simulink model "wave_test_qpsk"  (R2017b)
settings: Solver=VariableStepAuto  StartTime=0.0  StopTime=10.0  RelTol=1e-3
undefined symbols (not defined in the file): ip, sdrqpsktx, usb
libraries: plutoradiolib x1, dspvision x1, plutoradioblksprivate x1, commutil2 x1, commdigbbndpm3 x1, commfilt2 x1
settings Model: Creator=root  LastModifiedBy=root

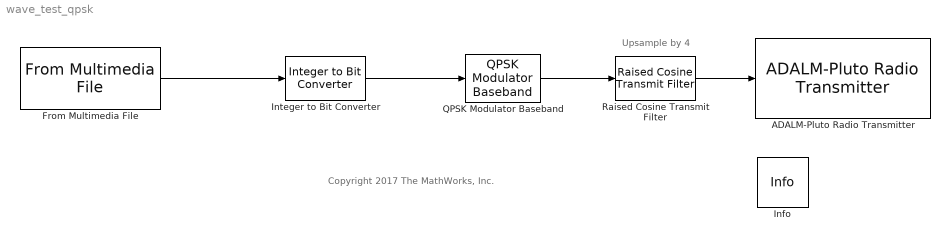
== system wave_test_qpsk ==
  note: Copyright 2017 The MathWorks, Inc.
  note: Upsample by 4
  ADALM-Pluto Radio Transmitter : plutoradiolib/ADALM-Pluto Radio Transmitter  SourceLibraryInfo="This block requires <a href=\"http://www.mathworks.com/hardware-support/rtl-sdr.html\">Communications System Toolbox Support Package for RTL-SDR Radio</a>"  RadioID=usb:0  uri=ip:10.0.0.200  CenterFrequencySource=Dialog  CenterFrequency=90.5e6  GainSource=Dialog  Gain=0  ChannelMapping=1  BasebandSampleRate=100e3  UnderflowOutputPort=off  ShowAdvancedProperties=off  Timeout=inf  DataSourceSelect=Input Port  DDSTone1Freq=5e3  DDSTone2Freq=10e3  DDSTone1Scale=0.5  DDSTone2Scale=0.25  FrequencyCorrection=0  UseCustomFilter=off  filtPathRates=[ 737280000, 11520000, 3840000, 1920000, 960000, 240000 ]  filtCoefficients=round( fir1( 127, 0.75 )*2^15*10^1.2 )  filtCoefficientSize=128  filtDecimInterpFactor=4  filtGain=-12  filtRFBandwidth=18e6  filterConfigStruct=struct()  ENSMPinControlMode=None  BISTLoopbackMode=Disabled
      settings: SourceProductName=Communications System Toolbox Support Package for ADALM-PLUTO Radio
  From Multimedia File : dspvision/From Multimedia File  inputFilename=/home/udsdrew/04_Let_Me_Be_Myself_mono.wav  loop=on  numPlays=inf  outputStreams=Audio only  videoDataType=single  audioDataType=int16  inheritSampleTime=on  userDefinedSampleTime=1/30  noAudioOutput=off  isIntensityVideo=off  fourcc=RGB  colorVideoFormat=One multidimensional signal  outputEOF=off  dataOrg=Column-major  audioFrameSize=8192  computeAudioFrameSize=off  outSamplingMode=Sample based
      settings: SourceProductBaseCode=VP
  Info : plutoradioblksprivate/Info  SystemSampleTime=-1
  Integer to Bit Converter : commutil2/Integer to Bit Converter  nbits=16  signedInputValues=Unsigned  bitOrder=MSB first  outDtype=Inherit via internal rule
  QPSK Modulator Baseband : commdigbbndpm3/QPSK Modulator Baseband  InType=Bit  Enc=Gray  Ph=pi/4  outDtype=double  outWordLen=16  outUDDataType=sfix(16)  outFracLenMode=Best precision  outFracLen=15  outDataTypeStr=double  outLastDataTypeStr=double
  Raised Cosine Transmit Filter : commfilt2/Raised Cosine Transmit Filter  filtType=Square root  R=sdrqpsktx.RollOff  filtSpan=sdrqpsktx.RCFiltSpan  N=sdrqpsktx.Upsampling  filterGain=1  InputProcessing=Columns as channels (frame based)  RateOptions=Enforce single-rate processing  framing=Mute  checkCoeff=off  variableName=rcTxFilt1  checkGain=Normalized  sampMode=Mute  saveAsFlag=0  currentFiltSpan=10  D=(sdrqpsktx.RCFiltSpan)/2  launchFVT=off  roundingMode=Floor  overflowMode=off  coeffDataTypeStr=Inherit: Same word length as input  coeffMin=[]  coeffMax=[]  coeffLastDataTypeStr=Inherit: Same word length as input  outputDataTypeStr=Inherit: Same as accumulator  outputMin=[]  outputMax=[]  outputLastDataTypeStr=Inherit: Same as accumulator
  wires:
  Raised Cosine Transmit Filter/1 -> ADALM-Pluto Radio Transmitter/1
  QPSK Modulator Baseband/1 -> Raised Cosine Transmit Filter/1
  From Multimedia File/1 -> Integer to Bit Converter/1
  Integer to Bit Converter/1 -> QPSK Modulator Baseband/1
